simulink model "VCU_SW"  (R2020b)
settings: Solver=FixedStepDiscrete  StartTime=0.0  StopTime=inf  FixedStep=1e-2  RelTol=1e-3
PreLoadFcn:
  | RTWConfigurationCB('preloadfcn', bdroot);
InitFcn:
  | loadvar_ttc500
undefined symbols (not defined in the file or in its folder): BrkPedalTypes, CabMovModeTypes, cFuseTempSensAcc_X, cFuseTempSensAcc_Y, cFuseTempSensVal_X, cFuseTempSensVal_Y, cTMSTempSensVal_X, cTMSTempSensVal_Y, cTransferCaseSpeedRatio, diag_state, DoorsPositionTypes, dP_filter_Y, DriverOccClassSystemTypes, ErrorValueTypes, fatal_error_callback, IO_ADC_NO_RANGE, LadderStatusTypes, pAnalogCabRotSensAcc, pAnalogCabRotSensMaxVolt, pAnalogCabRotSensMinVolt, pAnalogCabRotSensRange, pAnalogCabRotSensZeroVolt, pBrkActivePress, pCabTiltSensAcc, pCabTiltSensMaxCur, pCabTiltSensMinCur, pDistanceCorrection, pECANManual_BPNEnable, pECANManual_BPNEnabler_Flag, pFilterSensAccRes, pHDirMaxDiffFrq, pHDirSensHighLvl, pHDirSensLowLvl, pMainGearRatio, pMaxFilterSensRes, pMaxFirstPedalSensValue, pMaxFuseTempSensRes, pMaxPressLoss, pMaxPressSensCurrent, pMaxPressValue, pMaxPressValueHydMotAndPump, pMaxPressValueParkDrain, pMaxSecondPedalSensValue, pMaxTempSensVoltage, pMaxTempValue, pMaxTMSTempSensRes, pMinFilterSensRes, pMinFirstPedalSensValue, pMinFuseTempSensRes, pMinPressLoss, pMinPressSensCurrent, pMinPressValue, pMinSecondPedalSensValue, pMinTempSensVoltage, pMinTempValue, pMinTMSTempSensRes, pMotorRingTeethNum, pPedalSensAccuracyPct, pPedalSensAccuracyVolt, pPressLossTreshhold ... (+20)
libraries: TTlibrary x271, canmsglib x128, simulink x88
(part 14 of 17)

== system VCU_SW/InputLayer/InputInterfaces/AnalogInput/AIProc1000msec/TemperatureValues/calcFuseTemp ==
  note: Подумай как учесть погрешность без использования значения
      | с предыдущего шага
  calcFuseTemp : TriggerPort  TriggerType=function-call  IsSimulinkFunction=on  FunctionName=calcFuseTemp  FunctionVisibility=scoped  VariantControl=(inherit)
  Constant1 : Constant  Value=uint32(ErrorValueTypes.RESISTANSE_ERROR_VALUE)
  Constant2 : Constant  Value=int16(ErrorValueTypes.TEMPERATURE_ERROR_VALUE)
  Constant3 : Constant  Value=pMaxFuseTempSensRes
  Constant4 : Constant  Value=pMinFuseTempSensRes
  Data Type Conversion : DataTypeConversion  OutDataTypeStr=single
  Data Type Conversion1 : DataTypeConversion  OutDataTypeStr=int16
  Ground : Ground
  Multiport Switch : MultiPortSwitch  DataPortOrder=Zero-based contiguous  Inputs=2  zeroidx=on
  Relational Operator1 : RelationalOperator  Operator===  OutDataTypeStr='uint8'  RndMeth=Simplest
  Saturation Dynamic : simulink/Discontinuities/Saturation Dynamic  OutMin=[]  OutMax=[]  OutDataTypeStr=Inherit: Same as second input  OutDataType=fixdt(1, 16)  OutScaling=2^-10  DoSatur=off
  TempSensAccuracy : Lookup_n-D  NumberOfTableDimensions=1  BreakpointsForDimension1=cFuseTempSensAcc_X  Table=cFuseTempSensAcc_Y  ExtrapMethod=Clip  UseLastTableValue=on  InternalRulePriority=Speed  RndMeth=Simplest  InputSameDT=on
  TempSensValue : Lookup_n-D  NumberOfTableDimensions=1  BreakpointsForDimension1=cFuseTempSensVal_X  Table=cFuseTempSensVal_Y  ExtrapMethod=Clip  UseLastTableValue=on  InternalRulePriority=Speed  RndMeth=Simplest  InputSameDT=on
  Terminator : Terminator
  resistValue : ArgIn  DisableCoverage=on  OutDataTypeStr=uint32  ArgumentName=resistValue
  tempValue : ArgOut  DisableCoverage=on  OutDataTypeStr=int16  ArgumentName=tempValue
  wires:
  resistValue/1 -> Saturation Dynamic/2, Relational Operator1/2
  Relational Operator1/1 -> Multiport Switch/1
  Constant1/1 -> Relational Operator1/1
  Constant2/1 -> Multiport Switch/3
  Ground/1 -> TempSensAccuracy/1
  TempSensAccuracy/1 -> Terminator/1
  Data Type Conversion/1 -> TempSensValue/1
  TempSensValue/1 -> Data Type Conversion1/1
  Multiport Switch/1 -> tempValue/1
  Saturation Dynamic/1 -> Data Type Conversion/1
  Constant3/1 -> Saturation Dynamic/1
  Constant4/1 -> Saturation Dynamic/3
  Data Type Conversion1/1 -> Multiport Switch/2

== system VCU_SW/InputLayer/InputInterfaces/AnalogInput/AIProc1000msec/TemperatureValues/calcTMSTemp ==
  calcTMSTemp : TriggerPort  TriggerType=function-call  IsSimulinkFunction=on  FunctionName=calcTMSTemp  FunctionVisibility=scoped  VariantControl=(inherit)
  Constant : Constant  Value=uint32(ErrorValueTypes.RESISTANSE_ERROR_VALUE)
  Constant1 : Constant  Value=pMaxTMSTempSensRes
  Constant2 : Constant  Value=pMinTMSTempSensRes
  Constant3 : Constant  Value=int16(ErrorValueTypes.TEMPERATURE_ERROR_VALUE)
  Data Type Conversion : DataTypeConversion  OutDataTypeStr=single
  Data Type Conversion1 : DataTypeConversion  OutDataTypeStr=int16
  MATLAB Function : MATLAB Function  Commented=on  TreatAsAtomicUnit=on
  Multiport Switch1 : MultiPortSwitch  DataPortOrder=Zero-based contiguous  Inputs=2  zeroidx=on
  Relational Operator : RelationalOperator  Operator===  OutDataTypeStr='uint8'  RndMeth=Simplest
  Saturation Dynamic : simulink/Discontinuities/Saturation Dynamic  OutMin=[]  OutMax=[]  OutDataTypeStr=Inherit: Same as second input  OutDataType=fixdt(1, 16)  OutScaling=2^-10  DoSatur=off
  TempSensValue : Lookup_n-D  NumberOfTableDimensions=1  BreakpointsForDimension1=cTMSTempSensVal_X  IndexSearchMethod=Linear search  Table=cTMSTempSensVal_Y  ExtrapMethod=Clip  RemoveProtectionInput=on  UseLastTableValue=on  InternalRulePriority=Speed  OutDataTypeStr=Inherit: Inherit from 'Table data'  RndMeth=Round  InputSameDT=on
  customLookUpTableMF : MATLAB Function  Commented=on  TreatAsAtomicUnit=on
  resistValue : ArgIn  DisableCoverage=on  OutDataTypeStr=uint32  ArgumentName=resistValue
  tempValue : ArgOut  DisableCoverage=on  OutDataTypeStr=int16  ArgumentName=tempValue
  wires:
  Constant/1 -> Relational Operator/1
  Data Type Conversion/1 -> TempSensValue/1
  Constant3/1 -> Multiport Switch1/3
  Multiport Switch1/1 -> tempValue/1
  Constant2/1 -> Saturation Dynamic/3
  Saturation Dynamic/1 -> Data Type Conversion/1
  Constant1/1 -> Saturation Dynamic/1
  Relational Operator/1 -> Multiport Switch1/1
  resistValue/1 -> Saturation Dynamic/2, Relational Operator/2
  TempSensValue/1 -> Data Type Conversion1/1
  Data Type Conversion1/1 -> Multiport Switch1/2

== system VCU_SW/InputLayer/InputInterfaces/AnalogInput/AIProc100msec/PressureValues/calcCurPressSensVal ==
  calcCurPressSens : TriggerPort  TriggerType=function-call  IsSimulinkFunction=on  FunctionName=calcCurPressSens  FunctionVisibility=scoped  VariantControl=(inherit)
  Constant12 : Constant  Value=pPressSensAccCur
  Constant8 : Constant  Value=pMaxPressSensCurrent
  Constant9 : Constant  Value=pMinPressSensCurrent
  MATLAB Function : MATLAB Function  TreatAsAtomicUnit=on
  sensValue : ArgIn  DisableCoverage=on  OutDataTypeStr=uint16  ArgumentName=sensValue
  pressMax : ArgIn  Port=2  OutDataTypeStr=uint32  ArgumentName=pressMax
  pressMin : ArgIn  Port=3  OutDataTypeStr=uint32  ArgumentName=pressMin
  pressValue : ArgOut  DisableCoverage=on  OutDataTypeStr=uint32  ArgumentName=pressValue
  wires:
  MATLAB Function/1(pressureValue) -> pressValue/1
  Constant12/1 -> MATLAB Function/4(accuracyValue)
  pressMax/1 -> MATLAB Function/6(maxPress)
  pressMin/1 -> MATLAB Function/5(minPress)
  Constant8/1 -> MATLAB Function/1(maxValue)
  Constant9/1 -> MATLAB Function/2(minValue)
  sensValue/1 -> MATLAB Function/3(sensorValue)

== system VCU_SW/InputLayer/InputInterfaces/AnalogInput/AIProc10msec/CabMovValues/Simulink Function ==
  setPitchAngle : TriggerPort  TriggerType=function-call  IsSimulinkFunction=on  FunctionName=setPitchAngle  FunctionVisibility=scoped  VariantControl=(inherit)
  MATLAB Function1 : MATLAB Function  TreatAsAtomicUnit=on
  pitchSens : ArgIn  DisableCoverage=on  OutDataTypeStr=int16  ArgumentName=pitchSens
  pitchAngle : ArgOut  OutDataTypeStr=uint16  ArgumentName=pitchAngle
  pitchDir : ArgOut  Port=2  OutDataTypeStr=Enum: CabPitchDirTypes  ArgumentName=pitchDir
  wires:
  pitchSens/1 -> MATLAB Function1/1(cabTiltLongSens)
  MATLAB Function1/1(cabPitchAngle) -> pitchAngle/1
  MATLAB Function1/2(cabPitchAngleDir) -> pitchDir/1

== system VCU_SW/InputLayer/InputInterfaces/AnalogInput/AIProc10msec/CabMovValues/Simulink Function1 ==
  setRollAngle : TriggerPort  TriggerType=function-call  IsSimulinkFunction=on  FunctionName=setRollAngle  FunctionVisibility=scoped  VariantControl=(inherit)
  MATLAB Function2 : MATLAB Function  TreatAsAtomicUnit=on
  rollSens : ArgIn  DisableCoverage=on  OutDataTypeStr=int16  ArgumentName=rollSens
  rollAngle : ArgOut  OutDataTypeStr=uint16  ArgumentName=rollAngle
  rollDir : ArgOut  Port=2  OutDataTypeStr=Enum: CabRollDirTypes  ArgumentName=rollDir
  wires:
  rollSens/1 -> MATLAB Function2/1(cabTiltTransSens)
  MATLAB Function2/1(cabRollAngle) -> rollAngle/1
  MATLAB Function2/2(cabRollAngleDir) -> rollDir/1

== system VCU_SW/InputLayer/InputInterfaces/AnalogInput/AIProc10msec/CabMovValues/getAnalogCabRotSensData ==
  getAnalogCabRotSensData : TriggerPort  TriggerType=function-call  IsSimulinkFunction=on  FunctionName=getAnalogCabRotSensData  FunctionVisibility=scoped  VariantControl=(inherit)
  Constant1 : Constant  Value=pSlewDriveTransferRatio
  Constant2 : Constant  Value=pAnalogCabRotSensRange
  Constant3 : Constant  Value=pAnalogCabRotSensMaxVolt
  Constant4 : Constant  Value=pAnalogCabRotSensMinVolt
  Constant5 : Constant  Value=pAnalogCabRotSensAcc
  Constant6 : Constant  Value=pAnalogCabRotSensZeroVolt
  Data Store Read1 : DataStoreRead  DataStoreName=InputInterfaceData  DataStoreElements=InputInterfaceData.AI.rotCabAngleSens1
  Data Store Read2 : DataStoreRead  DataStoreName=InputInterfaceData  DataStoreElements=InputInterfaceData.AI.rotCabAngleSens2
  getAnalogCabRotSensData fcn : MATLAB Function  TreatAsAtomicUnit=on
  cabAngleCh1 : ArgOut  DisableCoverage=on  OutDataTypeStr=int16  ArgumentName=cabAngleCh1
  cabAngleCh2 : ArgOut  Port=2  OutDataTypeStr=int16  ArgumentName=cabAngleCh2
  wires:
  Data Store Read2/1 -> getAnalogCabRotSensData fcn/2(voltCh2)
  Data Store Read1/1 -> getAnalogCabRotSensData fcn/1(voltCh1)
  getAnalogCabRotSensData fcn/1(cabAngleCh1) -> cabAngleCh1/1
  getAnalogCabRotSensData fcn/2(cabAngleCh2) -> cabAngleCh2/1
  Constant2/1 -> getAnalogCabRotSensData fcn/3(sensRange)
  Constant1/1 -> getAnalogCabRotSensData fcn/8(transferRatio)
  Constant4/1 -> getAnalogCabRotSensData fcn/5(minVolt)
  Constant5/1 -> getAnalogCabRotSensData fcn/7(accuracy)
  Constant6/1 -> getAnalogCabRotSensData fcn/6(zeroVolt)
  Constant3/1 -> getAnalogCabRotSensData fcn/4(maxVolt)

== system VCU_SW/InputLayer/InputInterfaces/AnalogInput/AIProc10msec/CabMovValues/getCabTiltSensData ==
  getSensData : TriggerPort  TriggerType=function-call  IsSimulinkFunction=on  FunctionName=getSensData  FunctionVisibility=scoped  VariantControl=(inherit)
  Function Caller : FunctionCaller  FunctionPrototype=cabTiltAngle = cabTiltSensProc(rawCur)  InputArgumentSpecifications=<Enter example>  OutputArgumentSpecifications=<Enter example>
  Function Caller1 : FunctionCaller  FunctionPrototype=cabTiltAngle = cabTiltSensProc(rawCur)  InputArgumentSpecifications=<Enter example>  OutputArgumentSpecifications=<Enter example>
  Simulink Function : Subsystem  TreatAsAtomicUnit=on
  pitchAngleSens : ArgIn  OutDataTypeStr=uint16  ArgumentName=pitchAngleSens
  rollAngleSens : ArgIn  Port=2  OutDataTypeStr=uint16  ArgumentName=rollAngleSens
  PitchAngle : ArgOut  DisableCoverage=on  OutDataTypeStr=int16  ArgumentName=PitchAngle
  RollAngle : ArgOut  Port=2  OutDataTypeStr=int16  ArgumentName=RollAngle
  wires:
  rollAngleSens/1 -> Function Caller1/1
  pitchAngleSens/1 -> Function Caller/1
  Function Caller/1 -> PitchAngle/1
  Function Caller1/1 -> RollAngle/1

== system VCU_SW/InputLayer/InputInterfaces/AnalogInput/AIProc10msec/CabMovValues/setAnalogCabRotSensData ==
  setAnalogCabRotSensData : TriggerPort  TriggerType=function-call  IsSimulinkFunction=on  FunctionName=setAnalogCabRotSensData  FunctionVisibility=scoped  VariantControl=(inherit)
  Data Store Write1 : DataStoreWrite  DataStoreName=InputFunctionsData  DataStoreElements=InputFunctionsData.rotCabAngleValue
  Data Store Write2 : DataStoreWrite  DataStoreName=InputFunctionsData  DataStoreElements=InputFunctionsData.rotCabAngleDir
  cabRotSensConv fcn : MATLAB Function  TreatAsAtomicUnit=on
  cabAngleCh1 : ArgIn  DisableCoverage=on  OutDataTypeStr=int16  ArgumentName=cabAngleCh1
  cabAngleCh2 : ArgIn  Port=2  OutDataTypeStr=int16  ArgumentName=cabAngleCh2
  wires:
  cabAngleCh1/1 -> cabRotSensConv fcn/1(cabAngleCh1)
  cabAngleCh2/1 -> cabRotSensConv fcn/2(cabAngleCh2)
  cabRotSensConv fcn/1(cabAngle) -> Data Store Write1/1
  cabRotSensConv fcn/2(cabAngleDir) -> Data Store Write2/1

== system VCU_SW/InputLayer/InputInterfaces/AnalogInput/AIProc10msec/CabMovValues/setAnalogSensErr ==
  setAnalogSensErr : TriggerPort  TriggerType=function-call  IsSimulinkFunction=on  FunctionName=setAnalogSensErr  FunctionVisibility=scoped  VariantControl=(inherit)
  Data Store Write1 : DataStoreWrite  DataStoreName=InputFunctionsData  DataStoreElements=InputFunctionsData.cabRotAnalogSensErr
  err : ArgIn  DisableCoverage=on  OutDataTypeStr=boolean  ArgumentName=err
  wires:
  err/1 -> Data Store Write1/1

== system VCU_SW/InputLayer/InputInterfaces/AnalogInput/AIProc10msec/CabMovValues/setCabTiltSensData ==
  setCabTiltSensData : TriggerPort  TriggerType=function-call  IsSimulinkFunction=on  FunctionName=setCabTiltSensData  FunctionVisibility=scoped  VariantControl=(inherit)
  Data Store Write14 : DataStoreWrite  DataStoreName=UDSStruct  DataStoreElements=UDSStruct.cabTiltLeftLongSens
  Data Store Write15 : DataStoreWrite  DataStoreName=UDSStruct  DataStoreElements=UDSStruct.cabTiltLeftTransSens
  Data Store Write3 : DataStoreWrite  DataStoreName=InputFunctionsData  DataStoreElements=InputFunctionsData.cabPitchAngleValue
  Data Store Write4 : DataStoreWrite  DataStoreName=InputFunctionsData  DataStoreElements=InputFunctionsData.cabPitchAngleDir
  Data Store Write5 : DataStoreWrite  DataStoreName=InputFunctionsData  DataStoreElements=InputFunctionsData.cabRollAngleValue
  Data Store Write6 : DataStoreWrite  DataStoreName=InputFunctionsData  DataStoreElements=InputFunctionsData.cabRollAngleDir
  Function Caller : FunctionCaller  FunctionPrototype=[pitchAngle,pitchDir] = setPitchAngle(pitchSens)  InputArgumentSpecifications=<Enter example>  OutputArgumentSpecifications=<Enter example>
  Function Caller2 : FunctionCaller  FunctionPrototype=[rollAngle,rollDir] = setRollAngle(rollSens)  InputArgumentSpecifications=<Enter example>  OutputArgumentSpecifications=<Enter example>
  cabPitchAngle : ArgIn  OutDataTypeStr=int16  ArgumentName=cabPitchAngle
  cabRollAngle : ArgIn  Port=2  OutDataTypeStr=int16  ArgumentName=cabRollAngle
  wires:
  Function Caller2/1 -> Data Store Write5/1, Data Store Write15/1
  Function Caller/1 -> Data Store Write3/1, Data Store Write14/1
  cabPitchAngle/1 -> Function Caller/1
  cabRollAngle/1 -> Function Caller2/1
  Function Caller/2 -> Data Store Write4/1
  Function Caller2/2 -> Data Store Write6/1

== system VCU_SW/InputLayer/InputInterfaces/AnalogInput/AIProc10msec/CabMovValues/setCabTiltSensErr ==
  setCabTiltSensErr : TriggerPort  TriggerType=function-call  IsSimulinkFunction=on  FunctionName=setCabTiltSensErr  FunctionVisibility=scoped  VariantControl=(inherit)
  Data Store Write3 : DataStoreWrite  DataStoreName=InputFunctionsData  DataStoreElements=InputFunctionsData.cabTiltSensErr
  err : ArgIn  DisableCoverage=on  OutDataTypeStr=boolean  ArgumentName=err
  wires:
  err/1 -> Data Store Write3/1

== system VCU_SW/InputLayer/InputInterfaces/AnalogInput/AIProc10msec/CabMovValues/setFrameTiltSensData ==
  setFrameTiltSensData : TriggerPort  TriggerType=function-call  IsSimulinkFunction=on  FunctionName=setFrameTiltSensData  FunctionVisibility=scoped  VariantControl=(inherit)
  Data Store Write10 : DataStoreWrite  DataStoreName=InputFunctionsData  DataStoreElements=InputFunctionsData.frameRollAngleDir
  Data Store Write23 : DataStoreWrite  DataStoreName=UDSStruct  DataStoreElements=UDSStruct.longitudinalTransPlatfAngleSens
  Data Store Write26 : DataStoreWrite  DataStoreName=UDSStruct  DataStoreElements=UDSStruct.transverseTransPlatfAngleSens
  Data Store Write7 : DataStoreWrite  DataStoreName=InputFunctionsData  DataStoreElements=InputFunctionsData.framePitchAngleValue
  Data Store Write8 : DataStoreWrite  DataStoreName=InputFunctionsData  DataStoreElements=InputFunctionsData.framePitchAngleDir
  Data Store Write9 : DataStoreWrite  DataStoreName=InputFunctionsData  DataStoreElements=InputFunctionsData.frameRollAngleValue
  Function Caller1 : FunctionCaller  FunctionPrototype=[pitchAngle,pitchDir] = setPitchAngle(pitchSens)  InputArgumentSpecifications=<Enter example>  OutputArgumentSpecifications=<Enter example>
  Function Caller3 : FunctionCaller  FunctionPrototype=[rollAngle,rollDir] = setRollAngle(rollSens)  InputArgumentSpecifications=<Enter example>  OutputArgumentSpecifications=<Enter example>
  hullPitchAngle : ArgIn  OutDataTypeStr=int16  ArgumentName=hullPitchAngle
  hullRollAngle : ArgIn  Port=2  OutDataTypeStr=int16  ArgumentName=hullRollAngle
  wires:
  Function Caller3/1 -> Data Store Write9/1, Data Store Write26/1
  Function Caller1/1 -> Data Store Write7/1, Data Store Write23/1
  Function Caller3/2 -> Data Store Write10/1
  Function Caller1/2 -> Data Store Write8/1
  hullRollAngle/1 -> Function Caller3/1
  hullPitchAngle/1 -> Function Caller1/1

== system VCU_SW/InputLayer/InputInterfaces/AnalogInput/AIProc10msec/CabMovValues/setFrameTiltSensErr ==
  setFrameTiltSensErr : TriggerPort  TriggerType=function-call  IsSimulinkFunction=on  FunctionName=setFrameTiltSensErr  FunctionVisibility=scoped  VariantControl=(inherit)
  Data Store Write3 : DataStoreWrite  DataStoreName=InputFunctionsData  DataStoreElements=InputFunctionsData.frameTiltSensErr
  err : ArgIn  DisableCoverage=on  OutDataTypeStr=boolean  ArgumentName=err
  wires:
  err/1 -> Data Store Write3/1

== system VCU_SW/InputLayer/InputInterfaces/AnalogInput/AIProc10msec/PedalValues/calcPedalSensDirect ==
  calcPedalSensValue : TriggerPort  TriggerType=function-call  IsSimulinkFunction=on  FunctionName=calcPedalSensValue  FunctionVisibility=scoped  VariantControl=(inherit)
  Constant2 : Constant  Value=pPedalSensAccuracyVolt
  MATLAB Function : MATLAB Function  TreatAsAtomicUnit=on
  voltValue : ArgIn  OutDataTypeStr=uint16  ArgumentName=voltValue
  minValue : ArgIn  Port=2  OutDataTypeStr=uint16  ArgumentName=minValue
  maxValue : ArgIn  Port=3  OutDataTypeStr=uint16  ArgumentName=maxValue
  pctValue : ArgOut  DisableCoverage=on  OutDataTypeStr=uint8  ArgumentName=pctValue
  wires:
  MATLAB Function/1(pedalValue) -> pctValue/1
  voltValue/1 -> MATLAB Function/3(sensorValue)
  Constant2/1 -> MATLAB Function/4(accuracyValue)
  minValue/1 -> MATLAB Function/2(minValue)
  maxValue/1 -> MATLAB Function/1(maxValue)

== system VCU_SW/InputLayer/InputInterfaces/AnalogInput/AIProc10msec/PedalValues/validatePedalSensValue ==
  validatePedalSensValue : TriggerPort  TriggerType=function-call  IsSimulinkFunction=on  FunctionName=validatePedalSensValue  FunctionVisibility=scoped  VariantControl=(inherit)
  Constant : Constant  Value=pPedalSensAccuracyPct
  Ground : Ground
  MATLAB Function : MATLAB Function  TreatAsAtomicUnit=on
  fstValue : ArgIn  DisableCoverage=on  OutDataTypeStr=uint8  ArgumentName=fstValue
  secValue : ArgIn  Port=2  OutDataTypeStr=uint8  ArgumentName=secValue
  pedalVal : ArgOut  OutDataTypeStr=uint8  ArgumentName=pedalVal
  pedalVal1 : ArgOut  Port=2  OutDataTypeStr=uint8  ArgumentName=errorSts
  wires:
  MATLAB Function/1(pedalValue) -> pedalVal/1
  Ground/1 -> pedalVal1/1
  Constant/1 -> MATLAB Function/3(accuracyValue)
  secValue/1 -> MATLAB Function/2(secondSensValue)
  fstValue/1 -> MATLAB Function/1(firstSensValue)

== system VCU_SW/InputLayer/InputInterfaces/AnalogInput/AIProc10msec/PressureValues/Simulink Function ==
  brkPressFBproc : TriggerPort  TriggerType=function-call  IsSimulinkFunction=on  FunctionName=brkPressFBproc  FunctionVisibility=scoped  VariantControl=(inherit)
  MATLAB Function : MATLAB Function  TreatAsAtomicUnit=on
  pBrkActivePress : ArgIn  DisableCoverage=on  OutDataTypeStr=uint32  ArgumentName=pBrkActivePress
  pressFB : ArgIn  Port=2  OutDataTypeStr=uint32  ArgumentName=pressFB
  stt : ArgOut  DisableCoverage=on  OutDataTypeStr=Enum: StateModeTypes  ArgumentName=stt
  wires:
  MATLAB Function/1(stt) -> stt/1
  pressFB/1 -> MATLAB Function/2(pressFB)
  pBrkActivePress/1 -> MATLAB Function/1(pBrkActivePress)

== system VCU_SW/InputLayer/InputInterfaces/AnalogInput/AIProc10msec/PressureValues/calcCurPressSensVal ==
  calcCurPressSens : TriggerPort  TriggerType=function-call  IsSimulinkFunction=on  FunctionName=calcCurPressSens  FunctionVisibility=scoped  VariantControl=(inherit)
  Constant12 : Constant  Value=pPressSensAccCur
  Constant8 : Constant  Value=pMaxPressSensCurrent
  Constant9 : Constant  Value=pMinPressSensCurrent
  MATLAB Function : MATLAB Function  TreatAsAtomicUnit=on
  sensValue : ArgIn  DisableCoverage=on  OutDataTypeStr=uint16  ArgumentName=sensValue
  pressMax : ArgIn  Port=2  OutDataTypeStr=uint32  ArgumentName=pressMax
  pressMin : ArgIn  Port=3  OutDataTypeStr=uint32  ArgumentName=pressMin
  pressValue : ArgOut  DisableCoverage=on  OutDataTypeStr=uint32  ArgumentName=pressValue
  wires:
  sensValue/1 -> MATLAB Function/3(sensorValue)
  Constant9/1 -> MATLAB Function/2(minValue)
  Constant8/1 -> MATLAB Function/1(maxValue)
  pressMin/1 -> MATLAB Function/5(minPress)
  pressMax/1 -> MATLAB Function/6(maxPress)
  Constant12/1 -> MATLAB Function/4(accuracyValue)
  MATLAB Function/1(pressureValue) -> pressValue/1

== system VCU_SW/InputLayer/InputInterfaces/AnalogInput/AIProc10msec/PumpMotorDirections/calcRotDirSens ==
  calcRotDirSens : TriggerPort  TriggerType=function-call  IsSimulinkFunction=on  FunctionName=calcRotDirSens  FunctionVisibility=scoped  VariantControl=(inherit)
  Constant1 : Constant  Value=pHDirMaxDiffFrq
  Constant12 : Constant  Value=pHDirSensLowLvl
  Constant14 : Constant  Value=pHDirSensHighLvl
  MATLAB Function : MATLAB Function  TreatAsAtomicUnit=on
  sensValue : ArgIn  DisableCoverage=on  OutDataTypeStr=uint16  ArgumentName=sensValue
  SpdSensSig1 : ArgIn  Port=2  OutDataTypeStr=uint16  ArgumentName=SpdSensSig1
  SpdSensSig2 : ArgIn  Port=3  OutDataTypeStr=uint16  ArgumentName=SpdSensSig2
  RotDir : ArgOut  DisableCoverage=on  OutDataTypeStr=Enum: HydroAgrRotDirTypes  ArgumentName=RotDir
  wires:
  sensValue/1 -> MATLAB Function/3(sensorValue)
  Constant14/1 -> MATLAB Function/1(HighLvl)
  Constant12/1 -> MATLAB Function/2(LowLvl)
  MATLAB Function/1(RotDir) -> RotDir/1
  SpdSensSig2/1 -> MATLAB Function/6(SpdSensSig2)
  SpdSensSig1/1 -> MATLAB Function/5(SpdSensSig1)
  Constant1/1 -> MATLAB Function/4(MaxDiffFrq)

== system VCU_SW/InputLayer/InputInterfaces/DigitalInput/Function-Call Subsystem/cabRotIndSensProc/getIndRotSensData ==
  getIndRotSensData : TriggerPort  TriggerType=function-call  IsSimulinkFunction=on  FunctionName=getIndRotSensData  FunctionVisibility=scoped  VariantControl=(inherit)
  Data Store Read : DataStoreRead  DataStoreName=InputInterfaceData  DataStoreElements=InputInterfaceData.DI.extrLeftCabPosSens#InputInterfaceData.DI.extrRightCabPosSens
  getIndRotSensData fcn : MATLAB Function  TreatAsAtomicUnit=on
  getRotPos : Subsystem  TreatAsAtomicUnit=on
  cabRotPos : ArgOut  DisableCoverage=on  OutDataTypeStr=Enum: CabRotPosTypes  ArgumentName=cabRotPos
  wires:
  getIndRotSensData fcn/1(cabPos) -> cabRotPos/1
  Data Store Read/1 -> getIndRotSensData fcn/1(indSensLeft)
  Data Store Read/2 -> getIndRotSensData fcn/2(indSensRight)

== system VCU_SW/InputLayer/InputInterfaces/DigitalInput/Function-Call Subsystem/cabRotIndSensProc/setIndRotSensData ==
  setIndRotSensData : TriggerPort  TriggerType=function-call  IsSimulinkFunction=on  FunctionName=setIndRotSensData  FunctionVisibility=scoped  VariantControl=(inherit)
  Data Store Write2 : DataStoreWrite  DataStoreName=InputFunctionsData  DataStoreElements=InputFunctionsData.cabRotPos
  cabRotPos : ArgIn  DisableCoverage=on  OutDataTypeStr=Enum: CabRotPosTypes  ArgumentName=cabRotPos
  wires:
  cabRotPos/1 -> Data Store Write2/1

== system VCU_SW/InputLayer/InputInterfaces/DigitalInput/Function-Call Subsystem/cabRotIndSensProc/setIndSensErr ==
  setIndSensErr : TriggerPort  TriggerType=function-call  IsSimulinkFunction=on  FunctionName=setIndSensErr  FunctionVisibility=scoped  VariantControl=(inherit)
  Data Store Write3 : DataStoreWrite  DataStoreName=InputFunctionsData  DataStoreElements=InputFunctionsData.cabRotIndSensErr
  err : ArgIn  DisableCoverage=on  OutDataTypeStr=boolean  ArgumentName=err
  wires:
  err/1 -> Data Store Write3/1

== system VCU_SW/InputLayer/InputInterfaces/DigitalInput/Function-Call Subsystem2/cabRotIndSensProc/getIndRotSensData ==
  getIndRotSensData : TriggerPort  TriggerType=function-call  IsSimulinkFunction=on  FunctionName=getIndRotSensData  FunctionVisibility=scoped  VariantControl=(inherit)
  Data Store Read : DataStoreRead  DataStoreName=InputInterfaceData  DataStoreElements=InputInterfaceData.DI.extrLeftCabPosSens#InputInterfaceData.DI.extrRightCabPosSens
  getIndRotSensData fcn : MATLAB Function  TreatAsAtomicUnit=on
  getRotPos : Subsystem  TreatAsAtomicUnit=on
  cabRotPos : ArgOut  DisableCoverage=on  OutDataTypeStr=Enum: CabRotPosTypes  ArgumentName=cabRotPos
  wires:
  Data Store Read/2 -> getIndRotSensData fcn/1(indSensRight)
  Data Store Read/1 -> ?
  getIndRotSensData fcn/1(cabPos) -> cabRotPos/1

== system VCU_SW/InputLayer/InputInterfaces/DigitalInput/Function-Call Subsystem2/cabRotIndSensProc/setIndRotSensData ==
  setIndRotSensData : TriggerPort  TriggerType=function-call  IsSimulinkFunction=on  FunctionName=setIndRotSensData  FunctionVisibility=scoped  VariantControl=(inherit)
  Data Store Write2 : DataStoreWrite  DataStoreName=InputFunctionsData  DataStoreElements=InputFunctionsData.cabRotPos
  cabRotPos : ArgIn  DisableCoverage=on  OutDataTypeStr=Enum: CabRotPosTypes  ArgumentName=cabRotPos
  wires:
  cabRotPos/1 -> Data Store Write2/1

== system VCU_SW/InputLayer/InputInterfaces/DigitalInput/Function-Call Subsystem2/cabRotIndSensProc/setIndSensErr ==
  setIndSensErr : TriggerPort  TriggerType=function-call  IsSimulinkFunction=on  FunctionName=setIndSensErr  FunctionVisibility=scoped  VariantControl=(inherit)
  Data Store Write3 : DataStoreWrite  DataStoreName=InputFunctionsData  DataStoreElements=InputFunctionsData.cabRotIndSensErr
  err : ArgIn  DisableCoverage=on  OutDataTypeStr=boolean  ArgumentName=err
  wires:
  err/1 -> Data Store Write3/1

== system VCU_SW/InputLayer/InputNetwork/InputCCAN/CCAN100msecProc1/CabMov buttons processing/callRotFcn ==
  callRotFcn : TriggerPort  TriggerType=function-call  IsSimulinkFunction=on  FunctionName=callRotFcn  FunctionVisibility=scoped  VariantControl=(inherit)
  RotFcn : MATLAB Function  TreatAsAtomicUnit=on
  Subsystem : Subsystem
  Subsystem1 : Subsystem
  rotReturnAchieved : Subsystem  TreatAsAtomicUnit=on
  setReturnBut : Subsystem  TreatAsAtomicUnit=on
  rotState : ArgOut  OutDataTypeStr=Enum: CabMovModeTypes  ArgumentName=rotState
  wires:
  RotFcn/1(rotState) -> rotState/1
  Subsystem/1(rotReturnTrigger) -> RotFcn/1(rotReturnTrigger)
  Subsystem1/1(manualRotReq) -> RotFcn/2(manualRotReq)

== system VCU_SW/InputLayer/InputNetwork/InputCCAN/CCAN100msecProc1/CabMov buttons processing/callTiltFcn ==
  callTiltFcn : TriggerPort  TriggerType=function-call  IsSimulinkFunction=on  FunctionName=callTiltFcn  FunctionVisibility=scoped  VariantControl=(inherit)
  Subsystem : Subsystem
  Subsystem1 : Subsystem
  Subsystem2 : Subsystem
  TiltFcn : MATLAB Function  TreatAsAtomicUnit=on
  monkeyPressTilt : Subsystem  TreatAsAtomicUnit=on
  setAutoTiltBut : Subsystem  TreatAsAtomicUnit=on
  setTiltBut : Subsystem  TreatAsAtomicUnit=on
  tiltReturnAchieved : Subsystem  TreatAsAtomicUnit=on
  rotState : ArgIn  OutDataTypeStr=Enum: CabMovModeTypes  ArgumentName=rotState
  wires:
  rotState/1 -> TiltFcn/1(rotState)
  Subsystem/1(stabButTrigger) -> TiltFcn/2(stabButTrigger)
  Subsystem1/1(tiltReturnTrigger) -> TiltFcn/3(tiltReturnTrigger)
  Subsystem2/1(tiltPress) -> TiltFcn/4(tiltPress)

== system VCU_SW/InputLayer/InputNetwork/InputCCAN/CCAN100msecProc1/InputTransSelect/calcLeverPos ==
  calcLeverPos : TriggerPort  TriggerType=function-call  IsSimulinkFunction=on  FunctionName=calcLeverPos  FunctionVisibility=scoped  VariantControl=(inherit)
  MATLAB Function : MATLAB Function  TreatAsAtomicUnit=on
  TransReqGear : ArgIn  DisableCoverage=on  OutDataTypeStr=Enum: LeverPosTypes  ArgumentName=TransReqGear
  SelSig1 : ArgIn  Port=2  OutDataTypeStr=Enum: StateModeTypes  ArgumentName=SelSig1
  SelSig2 : ArgIn  Port=3  OutDataTypeStr=Enum: StateModeTypes  ArgumentName=SelSig2
  SelSig3 : ArgIn  Port=4  OutDataTypeStr=Enum: StateModeTypes  ArgumentName=SelSig3
  LeverPos : ArgOut  DisableCoverage=on  OutDataTypeStr=Enum: LeverPosTypes  ArgumentName=LeverPos
  wires:
  SelSig3/1 -> MATLAB Function/4(SelSig3)
  SelSig2/1 -> MATLAB Function/3(SelSig2)
  SelSig1/1 -> MATLAB Function/2(SelSig1)
  MATLAB Function/1(LeverPos) -> LeverPos/1
  TransReqGear/1 -> MATLAB Function/1(TransReqGear)

== system VCU_SW/OutputLayer/OutputNetwork/OutputDiagCAN + Logger/SetDiagCAN10msec/Simulink Function/Simulink Function2 ==
  parsingUDS : TriggerPort  TriggerType=function-call  IsSimulinkFunction=on  FunctionName=getNegMess  FunctionVisibility=scoped  VariantControl=(inherit)
  CANPack_UDS : canmsglib/CAN Pack  MsgList=(none)  MsgName=UDS  MsgIDType=Extended (29-bit identifier)  MsgIdentifier=215619578  MsgLength=8  Remote=off  ApplyMinMax=off  BusOutput=on  SignalInfo={ 'negative_id', '0', '8', 'LE', 'unsigned', 'Standard', '0', '1', '0', '0', '255'; 'service_id', '8', '8', 'LE', 'unsigned', 'Standard', '0', '1', '0', '0', '255'; 'NRC', '16', '8', 'LE', 'unsigned', 'Standard', '0', '1', '0', '0', '255' }
      settings: SourceProductBaseCode=ME,XP,VN  DataFormat=manually specified signals
  Terminator : Terminator
  transmit_message_dcdc_in_control : TTlibrary/CAN/transmit_message_name  channel=IO_CAN_CHANNEL_0  id_format=IO_CAN_EXT_FRAME  retranslation=off  io_error=on  sample_time=-1
      settings: SourceProductName=TT control 500 series
  service_id : ArgIn  DisableCoverage=on  OutDataTypeStr=uint8  ArgumentName=NegRes
  data_id : ArgIn  DisableCoverage=on  Port=2  OutDataTypeStr=uint8  ArgumentName=service_id
  data : ArgIn  DisableCoverage=on  Port=3  OutDataTypeStr=uint8  ArgumentName=NRC
  wires:
  CANPack_UDS/1 -> transmit_message_dcdc_in_control/1
  transmit_message_dcdc_in_control/1 -> Terminator/1  "error_tx_transmit_message_dcdc_in_control"
  service_id/1 -> CANPack_UDS/1
  data/1 -> CANPack_UDS/3
  data_id/1 -> CANPack_UDS/2

== system VCU_SW/OutputLayer/OutputNetwork/OutputDiagCAN + Logger/SetDiagCAN10msec/Simulink Function/Simulink Function3 ==
  getPosMess : TriggerPort  TriggerType=function-call  IsSimulinkFunction=on  FunctionName=getPosMess  FunctionVisibility=scoped  VariantControl=(inherit)
  CANPack_UDS : canmsglib/CAN Pack  MsgList=(none)  MsgName=UDS  MsgIDType=Extended (29-bit identifier)  MsgIdentifier=215619578  MsgLength=8  Remote=off  ApplyMinMax=off  BusOutput=on  SignalInfo={ 'Service_id', '0', '8', 'LE', 'unsigned', 'Standard', '0', '1', '0', '0', '255'; 'DataIdentifier', '8', '16', 'LE', 'unsigned', 'Standard', '0', '1', '0', '0', '65535'; 'DataRecord', '24', '16', 'LE', 'unsigned', 'Standard', '0', '1', '0', '0', '65535' }
      settings: SourceProductBaseCode=ME,XP,VN  DataFormat=manually specified signals
  Terminator : Terminator
  transmit_message_dcdc_in_control : TTlibrary/CAN/transmit_message_name  channel=IO_CAN_CHANNEL_1  id_format=IO_CAN_EXT_FRAME  retranslation=off  io_error=on  sample_time=-1
      settings: SourceProductName=TT control 500 series
  service_id : ArgIn  DisableCoverage=on  OutDataTypeStr=uint8  ArgumentName=service_id
  data_id : ArgIn  DisableCoverage=on  Port=2  OutDataTypeStr=uint16  ArgumentName=data_id
  data : ArgIn  DisableCoverage=on  Port=3  OutDataTypeStr=uint16  ArgumentName=data
  wires:
  CANPack_UDS/1 -> transmit_message_dcdc_in_control/1
  transmit_message_dcdc_in_control/1 -> Terminator/1  "error_tx_transmit_message_dcdc_in_control"
  service_id/1 -> CANPack_UDS/1
  data/1 -> CANPack_UDS/3
  data_id/1 -> CANPack_UDS/2

== system VCU_SW/OutputLayer/OutputNetwork/OutputDiagCAN + Logger/SetDiagCAN10msec1/Simulink Function/Simulink Function2 ==
  getNegMess : TriggerPort  TriggerType=function-call  IsSimulinkFunction=on  FunctionName=getNegMess  FunctionVisibility=scoped  VariantControl=(inherit)
  CANPack_UDS : canmsglib/CAN Pack  MsgList=(none)  MsgName=UDS  MsgIDType=Extended (29-bit identifier)  MsgIdentifier=215619578  MsgLength=8  Remote=off  ApplyMinMax=off  BusOutput=on  SignalInfo={ 'negative_id', '0', '8', 'LE', 'unsigned', 'Standard', '0', '1', '0', '0', '255'; 'service_id', '8', '8', 'LE', 'unsigned', 'Standard', '0', '1', '0', '0', '255'; 'NRC', '16', '8', 'LE', 'unsigned', 'Standard', '0', '1', '0', '0', '255' }
      settings: SourceProductBaseCode=ME,XP,VN  DataFormat=manually specified signals
  Terminator : Terminator
  transmit_message_dcdc_in_control : TTlibrary/CAN/transmit_message_name  channel=IO_CAN_CHANNEL_1  id_format=IO_CAN_EXT_FRAME  retranslation=off  io_error=on  sample_time=-1
      settings: SourceProductName=TT control 500 series
  NegRes : ArgIn  DisableCoverage=on  OutDataTypeStr=uint8  ArgumentName=NegRes
  service_id : ArgIn  DisableCoverage=on  Port=2  OutDataTypeStr=uint8  ArgumentName=service_id
  NRC : ArgIn  DisableCoverage=on  Port=3  OutDataTypeStr=uint8  ArgumentName=NRC
  wires:
  service_id/1 -> CANPack_UDS/2
  NRC/1 -> CANPack_UDS/3
  NegRes/1 -> CANPack_UDS/1
  transmit_message_dcdc_in_control/1 -> Terminator/1  "error_tx_transmit_message_dcdc_in_control"
  CANPack_UDS/1 -> transmit_message_dcdc_in_control/1

== system VCU_SW/OutputLayer/OutputNetwork/OutputDiagCAN + Logger/SetDiagCAN10msec1/Simulink Function/Simulink Function3 ==
  getPosMess : TriggerPort  TriggerType=function-call  IsSimulinkFunction=on  FunctionName=getPosMess  FunctionVisibility=scoped  VariantControl=(inherit)
  CANPack_UDS : canmsglib/CAN Pack  MsgList=(none)  MsgName=UDS  MsgIDType=Extended (29-bit identifier)  MsgIdentifier=215619578  MsgLength=8  Remote=off  ApplyMinMax=off  BusOutput=on  SignalInfo={ 'Service_id', '0', '8', 'LE', 'unsigned', 'Standard', '0', '1', '0', '0', '255'; 'DataIdentifier', '8', '16', 'LE', 'unsigned', 'Standard', '0', '1', '0', '0', '65535'; 'DataRecord', '24', '16', 'LE', 'unsigned', 'Standard', '0', '1', '0', '0', '65535' }
      settings: SourceProductBaseCode=ME,XP,VN  DataFormat=manually specified signals
  Terminator : Terminator
  transmit_message_dcdc_in_control : TTlibrary/CAN/transmit_message_name  channel=IO_CAN_CHANNEL_1  id_format=IO_CAN_EXT_FRAME  retranslation=off  io_error=on  sample_time=-1
      settings: SourceProductName=TT control 500 series
  service_id : ArgIn  DisableCoverage=on  OutDataTypeStr=uint8  ArgumentName=service_id
  data_id : ArgIn  DisableCoverage=on  Port=2  OutDataTypeStr=uint16  ArgumentName=data_id
  data : ArgIn  DisableCoverage=on  Port=3  OutDataTypeStr=uint16  ArgumentName=data
  wires:
  data_id/1 -> CANPack_UDS/2
  data/1 -> CANPack_UDS/3
  service_id/1 -> CANPack_UDS/1
  transmit_message_dcdc_in_control/1 -> Terminator/1  "error_tx_transmit_message_dcdc_in_control"
  CANPack_UDS/1 -> transmit_message_dcdc_in_control/1

== system VCU_SW/InputLayer/InputInterfaces/AnalogInput/AIProc10msec/CabMovValues/getCabTiltSensData/Simulink Function ==
  cabTiltSensProc : TriggerPort  TriggerType=function-call  IsSimulinkFunction=on  FunctionName=cabTiltSensProc  FunctionVisibility=scoped  VariantControl=(inherit)
  Constant1 : Constant  Value=pCabTiltSensMaxCur
  Constant2 : Constant  Value=pCabTiltSensMinCur
  Constant4 : Constant  Value=pCabTiltSensAcc
  MATLAB Function5 : MATLAB Function  TreatAsAtomicUnit=on
  rawCur : ArgIn  DisableCoverage=on  OutDataTypeStr=uint16  ArgumentName=rawCur
  cabTiltAngle : ArgOut  DisableCoverage=on  OutDataTypeStr=int16  ArgumentName=cabTiltAngle
  wires:
  Constant4/1 -> MATLAB Function5/4(accuracy)
  Constant1/1 -> MATLAB Function5/3(maxCur)
  Constant2/1 -> MATLAB Function5/2(minCur)
  rawCur/1 -> MATLAB Function5/1(cabTiltSens)
  MATLAB Function5/1(signedCabTiltAngle) -> cabTiltAngle/1

== system VCU_SW/InputLayer/InputInterfaces/DigitalInput/Function-Call Subsystem/cabRotIndSensProc/getIndRotSensData/getRotPos ==
  getRotPos : TriggerPort  TriggerType=function-call  IsSimulinkFunction=on  FunctionName=getRotPos  FunctionVisibility=scoped  VariantControl=(inherit)
  Data Store Read3 : DataStoreRead  DataStoreName=InputFunctionsData  DataStoreElements=InputFunctionsData.cabRotPos
  result : ArgOut  DisableCoverage=on  OutDataTypeStr=Enum: CabRotPosTypes  ArgumentName=result
  wires:
  Data Store Read3/1 -> result/1

== system VCU_SW/InputLayer/InputInterfaces/DigitalInput/Function-Call Subsystem2/cabRotIndSensProc/getIndRotSensData/getRotPos ==
  getRotPos : TriggerPort  TriggerType=function-call  IsSimulinkFunction=on  FunctionName=getRotPos  FunctionVisibility=scoped  VariantControl=(inherit)
  Data Store Read3 : DataStoreRead  DataStoreName=InputFunctionsData  DataStoreElements=InputFunctionsData.cabRotPos
  result : ArgOut  DisableCoverage=on  OutDataTypeStr=Enum: CabRotPosTypes  ArgumentName=result
  wires:
  Data Store Read3/1 -> result/1

== system VCU_SW/InputLayer/InputNetwork/InputCCAN/CCAN100msecProc1/CabMov buttons processing/callRotFcn/Subsystem ==
  AND : Logic  AllPortsSameDT=off  OutDataTypeStr=boolean
  Data Store Read4 : DataStoreRead  DataStoreName=InputNetworkData  DataStoreElements=InputNetworkData.CCAN.BJM1.But7CabRotReturn
  Enumerated Constant : simulink/Sources/Enumerated Constant  OutDataTypeStr=Enum: StateModeTypes  Value=StateModeTypes.STT_ENABLE  SampleTime=inf
  Enumerated Constant1 : simulink/Sources/Enumerated Constant  OutDataTypeStr=Enum: StateModeTypes  Value=StateModeTypes.STT_DISABLE  SampleTime=inf
  Relational Operator : RelationalOperator  Operator===  OutDataTypeStr=boolean  RndMeth=Simplest
  Relational Operator1 : RelationalOperator  Operator===  OutDataTypeStr=boolean  RndMeth=Simplest
  Unit Delay : UnitDelay  InitialCondition=StateModeTypes.STT_DISABLE  SampleTime=-1  HasFrameUpgradeWarning=on
  rotReturnTrigger : Outport
  wires:
  Data Store Read4/1 -> Unit Delay/1, Relational Operator/1
  Enumerated Constant/1 -> Relational Operator/2
  Enumerated Constant1/1 -> Relational Operator1/2
  Unit Delay/1 -> Relational Operator1/1
  Relational Operator/1 -> AND/1
  Relational Operator1/1 -> AND/2
  AND/1 -> rotReturnTrigger/1

== system VCU_SW/InputLayer/InputNetwork/InputCCAN/CCAN100msecProc1/CabMov buttons processing/callRotFcn/Subsystem1 ==
  Constant : Constant  Value=false
  Constant1 : Constant  Value=true
  Constant8 : Constant  Value=pRotCtrlThres
  Data Store Read3 : DataStoreRead  DataStoreName=InputFunctionsData  DataStoreElements=InputFunctionsData.rotJoyPos
  Data Type Conversion : DataTypeConversion  OutDataTypeStr=uint8
  Multiport Switch : MultiPortSwitch  DataPortOrder=Zero-based contiguous  Inputs=2  zeroidx=on
  Relational Operator : RelationalOperator  Operator=>  OutDataTypeStr=boolean  RndMeth=Simplest
  manualRotReq : Outport
  wires:
  Data Store Read3/1 -> Data Type Conversion/1
  Multiport Switch/1 -> manualRotReq/1
  Relational Operator/1 -> Multiport Switch/1
  Constant/1 -> Multiport Switch/2
  Constant1/1 -> Multiport Switch/3
  Constant8/1 -> Relational Operator/2
  Data Type Conversion/1 -> Relational Operator/1

== system VCU_SW/InputLayer/InputNetwork/InputCCAN/CCAN100msecProc1/CabMov buttons processing/callRotFcn/rotReturnAchieved ==
  rotReturnAchieved : TriggerPort  TriggerType=function-call  IsSimulinkFunction=on  FunctionName=rotReturnAchieved  FunctionVisibility=scoped  VariantControl=(inherit)
  Constant : Constant  Value=false
  Constant1 : Constant  Value=pRotAngleThres
  Constant2 : Constant  Value=true
  Data Store Read3 : DataStoreRead  DataStoreName=InputFunctionsData  DataStoreElements=InputFunctionsData.rotCabAngleValue
  Multiport Switch : MultiPortSwitch  DataPortOrder=Zero-based contiguous  Inputs=2  zeroidx=on
  Relational Operator1 : RelationalOperator  Operator=<=  OutDataTypeStr=boolean  RndMeth=Simplest
  rotState : ArgOut  OutDataTypeStr=boolean  ArgumentName=rotEnd
  wires:
  Constant1/1 -> Relational Operator1/2
  Data Store Read3/1 -> Relational Operator1/1
  Relational Operator1/1 -> Multiport Switch/1
  Multiport Switch/1 -> rotState/1
  Constant/1 -> Multiport Switch/2
  Constant2/1 -> Multiport Switch/3

== system VCU_SW/InputLayer/InputNetwork/InputCCAN/CCAN100msecProc1/CabMov buttons processing/callRotFcn/setReturnBut ==
  setReturnBut : TriggerPort  TriggerType=function-call  IsSimulinkFunction=on  FunctionName=setReturnBut  FunctionVisibility=scoped  VariantControl=(inherit)
  Data Store Write3 : DataStoreWrite  DataStoreName=InputFunctionsData  DataStoreElements=InputFunctionsData.exitBut
  butStt : ArgIn  OutDataTypeStr=Enum: StateModeTypes  ArgumentName=butStt
  wires:
  butStt/1 -> Data Store Write3/1

== system VCU_SW/InputLayer/InputNetwork/InputCCAN/CCAN100msecProc1/CabMov buttons processing/callTiltFcn/Subsystem ==
  AND : Logic  AllPortsSameDT=off  OutDataTypeStr=boolean
  Data Store Read4 : DataStoreRead  DataStoreName=InputNetworkData  DataStoreElements=InputNetworkData.CCAN.BJM1.But6CabStab
  Enumerated Constant : simulink/Sources/Enumerated Constant  OutDataTypeStr=Enum: StateModeTypes  Value=StateModeTypes.STT_ENABLE  SampleTime=inf
  Enumerated Constant1 : simulink/Sources/Enumerated Constant  OutDataTypeStr=Enum: StateModeTypes  Value=StateModeTypes.STT_DISABLE  SampleTime=inf
  Relational Operator : RelationalOperator  Operator===  OutDataTypeStr=boolean  RndMeth=Simplest
  Relational Operator1 : RelationalOperator  Operator===  OutDataTypeStr=boolean  RndMeth=Simplest
  Unit Delay : UnitDelay  InitialCondition=StateModeTypes.STT_DISABLE  SampleTime=-1  HasFrameUpgradeWarning=on
  stabButTrigger : Outport
  wires:
  Data Store Read4/1 -> Unit Delay/1, Relational Operator/1
  Enumerated Constant/1 -> Relational Operator/2
  Enumerated Constant1/1 -> Relational Operator1/2
  Unit Delay/1 -> Relational Operator1/1
  Relational Operator/1 -> AND/1
  Relational Operator1/1 -> AND/2
  AND/1 -> stabButTrigger/1

== system VCU_SW/InputLayer/InputNetwork/InputCCAN/CCAN100msecProc1/CabMov buttons processing/callTiltFcn/Subsystem1 ==
  AND : Logic  AllPortsSameDT=off  OutDataTypeStr=boolean
  Data Store Read4 : DataStoreRead  DataStoreName=InputNetworkData  DataStoreElements=InputNetworkData.CCAN.BJM1.But5CabTiltReturn
  Enumerated Constant : simulink/Sources/Enumerated Constant  OutDataTypeStr=Enum: StateModeTypes  Value=StateModeTypes.STT_ENABLE  SampleTime=inf
  Enumerated Constant1 : simulink/Sources/Enumerated Constant  OutDataTypeStr=Enum: StateModeTypes  Value=StateModeTypes.STT_DISABLE  SampleTime=inf
  Relational Operator : RelationalOperator  Operator===  OutDataTypeStr=boolean  RndMeth=Simplest
  Relational Operator1 : RelationalOperator  Operator===  OutDataTypeStr=boolean  RndMeth=Simplest
  Unit Delay : UnitDelay  InitialCondition=StateModeTypes.STT_DISABLE  SampleTime=-1  HasFrameUpgradeWarning=on
  tiltReturnTrigger : Outport
  wires:
  AND/1 -> tiltReturnTrigger/1
  Relational Operator1/1 -> AND/2
  Relational Operator/1 -> AND/1
  Unit Delay/1 -> Relational Operator1/1
  Enumerated Constant1/1 -> Relational Operator1/2
  Enumerated Constant/1 -> Relational Operator/2
  Data Store Read4/1 -> Relational Operator/1, Unit Delay/1

== system VCU_SW/InputLayer/InputNetwork/InputCCAN/CCAN100msecProc1/CabMov buttons processing/callTiltFcn/Subsystem2 ==
  Data Store Read1 : DataStoreRead  DataStoreName=InputNetworkData  DataStoreElements=InputNetworkData.CCAN.BJM1.But3CabPitchFwd
  Data Store Read2 : DataStoreRead  DataStoreName=InputNetworkData  DataStoreElements=InputNetworkData.CCAN.BJM1.But4CabPitchBckwd
  Data Store Read3 : DataStoreRead  DataStoreName=InputNetworkData  DataStoreElements=InputNetworkData.CCAN.BJM1.But2CabRollLeft
  Data Store Read4 : DataStoreRead  DataStoreName=InputNetworkData  DataStoreElements=InputNetworkData.CCAN.BJM1.But1CabRollRight
  Enumerated Constant{1..3,5} (4 alike) : simulink/Sources/Enumerated Constant  OutDataTypeStr=Enum: StateModeTypes  Value=StateModeTypes.STT_ENABLE  SampleTime=inf
  Logical Operator : Logic  Operator=OR  Inputs=4  AllPortsSameDT=off  OutDataTypeStr=boolean
  Relational Operator{,1..3} (4 alike) : RelationalOperator  Operator===  OutDataTypeStr=boolean  RndMeth=Simplest
  tiltPress : Outport
  wires:
  Logical Operator/1 -> tiltPress/1
  Data Store Read3/1 -> Relational Operator2/1
  Relational Operator1/1 -> Logical Operator/2
  Enumerated Constant5/1 -> Relational Operator/2
  Data Store Read2/1 -> Relational Operator1/1
  Enumerated Constant2/1 -> Relational Operator2/2
  Relational Operator2/1 -> Logical Operator/3
  Enumerated Constant1/1 -> Relational Operator1/2
  Data Store Read4/1 -> Relational Operator3/1
  Relational Operator3/1 -> Logical Operator/4
  Enumerated Constant3/1 -> Relational Operator3/2
  Relational Operator/1 -> Logical Operator/1

== system VCU_SW/InputLayer/InputNetwork/InputCCAN/CCAN100msecProc1/CabMov buttons processing/callTiltFcn/monkeyPressTilt ==
  monkeyPressTilt : TriggerPort  TriggerType=function-call  IsSimulinkFunction=on  FunctionName=monkeyPressTilt  FunctionVisibility=scoped  VariantControl=(inherit)
  Constant : Constant  Value=uint8(1)
  Constant1 : Constant  Value=true
  Constant2 : Constant  Value=false
  Data Store Read1 : DataStoreRead  DataStoreName=InputNetworkData  DataStoreElements=InputNetworkData.CCAN.BJM1.But3CabPitchFwd
  Data Store Read2 : DataStoreRead  DataStoreName=InputNetworkData  DataStoreElements=InputNetworkData.CCAN.BJM1.But4CabPitchBckwd
  Data Store Read3 : DataStoreRead  DataStoreName=InputNetworkData  DataStoreElements=InputNetworkData.CCAN.BJM1.But2CabRollLeft
  Data Store Read4 : DataStoreRead  DataStoreName=InputNetworkData  DataStoreElements=InputNetworkData.CCAN.BJM1.But1CabRollRight
  Data Type Conversion{,1..3} (4 alike) : DataTypeConversion  OutDataTypeStr=uint8
  Enumerated Constant{1..3,5} (4 alike) : simulink/Sources/Enumerated Constant  OutDataTypeStr=Enum: StateModeTypes  Value=StateModeTypes.STT_ENABLE  SampleTime=inf
  Multiport Switch : MultiPortSwitch  DataPortOrder=Zero-based contiguous  Inputs=2  zeroidx=on
  Relational Operator{,1..3} (4 alike) : RelationalOperator  Operator===  OutDataTypeStr=boolean  RndMeth=Simplest
  Relational Operator4 : RelationalOperator  Operator=>  OutDataTypeStr=boolean  RndMeth=Simplest
  Sum : Sum  Inputs=|++++
  result : ArgOut  OutDataTypeStr=boolean  ArgumentName=result
  wires:
  Multiport Switch/1 -> result/1
  Data Store Read1/1 -> Relational Operator/1
  Enumerated Constant5/1 -> Relational Operator/2
  Data Store Read2/1 -> Relational Operator1/1
  Enumerated Constant1/1 -> Relational Operator1/2
  Data Store Read3/1 -> Relational Operator2/1
  Enumerated Constant2/1 -> Relational Operator2/2
  Data Store Read4/1 -> Relational Operator3/1
  Enumerated Constant3/1 -> Relational Operator3/2
  Relational Operator/1 -> Data Type Conversion/1
  Relational Operator1/1 -> Data Type Conversion1/1
  Relational Operator2/1 -> Data Type Conversion2/1
  Relational Operator3/1 -> Data Type Conversion3/1
  Data Type Conversion/1 -> Sum/1
  Data Type Conversion1/1 -> Sum/2
  Data Type Conversion2/1 -> Sum/3
  Data Type Conversion3/1 -> Sum/4
  Sum/1 -> Relational Operator4/1
  Constant/1 -> Relational Operator4/2
  Relational Operator4/1 -> Multiport Switch/1
  Constant2/1 -> Multiport Switch/2
  Constant1/1 -> Multiport Switch/3
